simulink model "SF012A_HysCmp"  (R2013b)
settings: Solver=FixedStepDiscrete  StartTime=0.0  StopTime=1  FixedStep=.002  RelTol=1e-3
values from neighbouring files (symbols this model uses):
  ARCHGLBPRM_2MILLISEC_SEC_F32 = DataDict.Constant    [SF012A_HysCmp_DataDict.m]
  EPSILON_ULS_F32 = DataDict.Constant    [SF012A_HysCmp_DataDict.m]
  FLTINJ_HYSCMP_HYSCMPCMD = DataDict.Constant    [SF012A_HysCmp_DataDict.m]
  HysCmpAssiInpLim = DataDict.Calibration    [SF012A_HysCmp_DataDict.m]
  HysCmpOutpLim = DataDict.Calibration    [SF012A_HysCmp_DataDict.m]
  HysCmpRevGain = DataDict.Calibration    [SF012A_HysCmp_DataDict.m]
  HysCmpRiseX = DataDict.Calibration    [SF012A_HysCmp_DataDict.m]
  HysCmpRiseY = DataDict.Calibration    [SF012A_HysCmp_DataDict.m]
  HYSRISEYLIM_ULS_F32 = DataDict.Constant    [SF012A_HysCmp_DataDict.m]
  HYSSATNLOWLIM_HWNWTMTR_F32 = DataDict.Constant    [SF012A_HysCmp_DataDict.m]
  SysGlbPrmSysTqRat = DataDict.ImprtdCal    [SF012A_HysCmp_DataDict.m]
libraries: FixdToFloat x18, FloatToFixd x14, LnrIntrpn x12, NxtrAbslt x10, NxtrLim x8, Fil x6, NxtrSign x5, simulink x2, NxtrMath x1, BilnrIntrpnMplX x1, NxtrMax x1
(part 1 of 3)
settings Model: Creator=TZ5743  LastModifiedBy=NZ2883
settings DataIOCC: LimitDataPoints=off  SaveFormat=Structure  ReturnWorkspaceOutputs=on
settings OptimizationCC: BlockReduction=off  InlineParams=on  ZeroExternalMemoryAtStartup=off  ZeroInternalMemoryAtStartup=off  OptimizeModelRefInitCode=on  LifeSpan=1
settings DebuggingCC: SignalInfNanChecking=error  SignalRangeChecking=warning  UnderspecifiedInitializationDetection=Simplified  SolverPrmCheckMsg=error  InheritedTsInSrcMsg=error  DiscreteInheritContinuousMsg=error  SingleTaskRateTransMsg=error  TasksWithSamePriorityMsg=error  SigSpecEnsureSampleTimeMsg=error  CheckMatrixSingularityMsg=error  IntegerOverflowMsg=error  ParameterUnderflowMsg=error  ParameterPrecisionLossMsg=error  ParameterTunabilityLossMsg=error  FixptConstUnderflowMsg=warning  FixptConstOverflowMsg=warning  VectorMatrixConversionMsg=error  SignalLabelMismatchMsg=error  UnconnectedInputMsg=error  UnconnectedOutputMsg=error  UnconnectedLineMsg=error  SFcnCompatibilityMsg=error  UniqueDataStoreMsg=warning  BusObjectLabelMismatch=error  RootOutportRequireBusObject=error  AssertControl=DisableAll  ModelReferenceIOMsg=error  ModelReferenceVersionMismatchMessage=warning  ModelReferenceIOMismatchMessage=error  ModelReferenceCSMismatchMessage=warning  ModelReferenceDataLoggingMessage=error  StateNameClashWarn=warning  StrictBusMsg=ErrorOnBusTreatedAsVector  NonBusSignalsTreatedAsBus=error  SFUnexpectedBacktrackingDiag=error  SFInvalidInputDataAccessInChartInitDiag=error  SFNoUnconditionalDefaultTransitionDiag=error  SFTransitionOutsideNaturalParentDiag=error  SFUnconditionalTransitionShadowingDiag=error  SFUndirectedBroadcastEventsDiag=error
settings ModelReferenceCC: ModelReferenceNumInstancesAllowed=Single
settings RTWCC: SystemTargetFile=autosar.tlc  GenCodeOnly=on  TemplateMakefile=ert_default_tmf  Description=AUTOSAR  GenerateReport=on  ProcessScript=autosar_make_rtw_hook  LaunchReport=on
settings CodeAppCC: GenerateComments=off  IgnoreCustomStorageClasses=off  CustomSymbolStrType=$N$R$M  CustomSymbolStrBlkIO=$N$M  SimulinkBlockComments=off
settings STFCustomTargetCC: ParMdlRefBuildCompliant=on  CompOptLevelCompliant=on  IncludeMdlTerminateFcn=off  CombineOutputUpdateFcns=on  SuppressErrorStatus=on  ERTFirstTimeCompliant=on  ERTCustomFileBanners=on  SupportNonFinite=off  SupportComplex=off  SupportContinuousTime=off  SupportNonInlinedSFcns=off  MATLABClassNameForMDSCustomization=Simulink.SoftwareTarget.ERTCustomization  AutosarCompliant=on  GRTInterface=off  SystemTargetFile=autosar.tlc
settings ERTTargetCC: CodeReplacementLibrary=ANSI_C  ConcurrentExecutionCompliant=off  IncludeMdlTerminateFcn=off  SuppressErrorStatus=on  SupportNonFinite=off  SupportComplex=off  ModelStepFunctionPrototypeControlCompliant=off  CPPClassGenCompliant=off  AutosarCompliant=on  InlinedParameterPlacement=NonHierarchical  ERTCustomFileTemplate=example_file_process.tlc  EnableUserReplacementTypes=on

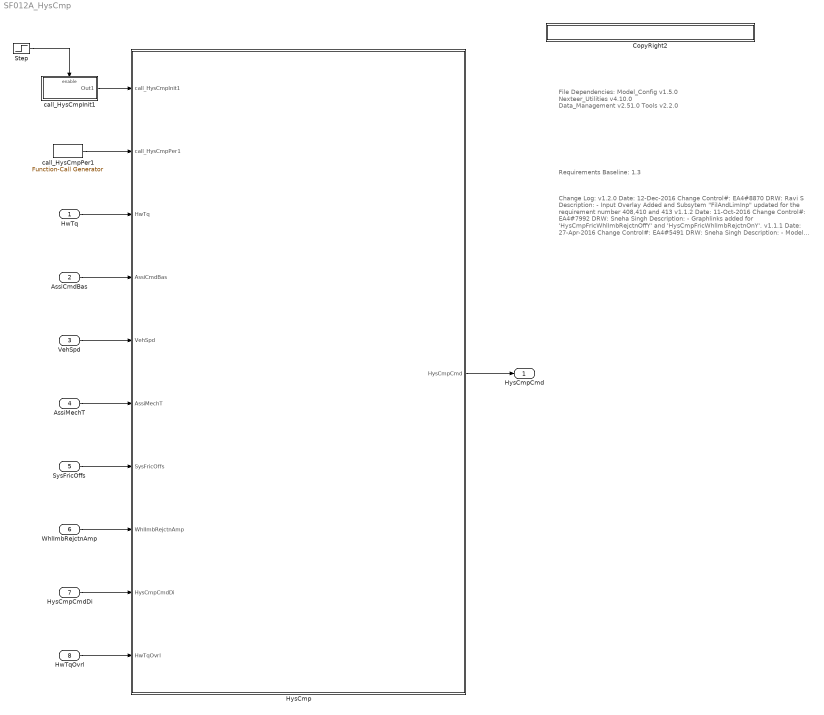
== system SF012A_HysCmp ==
  note: File Dependencies:
      |
      | Model_Config v1.5.0
      | Nexteer_Utilities v4.10.0
      | Data_Management v2.51.0
      | Tools v2.2.0
  note: Requirements Baseline: 1.3
  note: Change Log:
      |
      | v1.2.0
      | Date: 12-Dec-2016
      | Change Control#: EA4#8870
      | DRW: Ravi S
      | Description:
      | - Input Overlay Added and Subsytem "FilAndLimInp" updated
      |  for the requirement number 408,410 and 413
      |
      | v1.1.2
      | Date: 11-Oct-2016
      | Change Control#: EA4#7992
      | DRW: Sneha Singh
      | Description:
      | - Graphlinks added for 'HysCmpFricWhlImbRejctnOffY'
      | and 'HysCmpFricWhlImbRejctnOnY'.
      |
      | v1.1.1
      | Date: 27-Apr-2016
      | Change Control#: EA4#5491
      | DRW: Sneha Singh
      | Description:
      | - Model traceability performed in DOORS.
      |
      | v1.1.0
      | Date: 24-DEC-2015
      | Change Control #: EA4#2177
      | DRW:  Sumit/Muragesh(KPIT)
      | Description:
      | -  LPF block kept outside IF/ELSE Blocks from HysCmp.
      |
      | v1.0.0
      | Date: 08-Jul-2015
      | Change Control #: EA4#943
      | Author:  Sudeep Shankar
      | Description:
      | - Initial Release based off of EA3 Version 008
  HwTq : Inport  RequirementInfo={'linktype_rmi_doors' '0000a52c (/E-STEER Core/SubSystem Specifications/Application Functions/SF012A Hysteresis Compensation)' '#SF012A_393' 'true' 'REQ:SF012A_393' '' } %GIDa_39e8ddae_593d_4cef_93cb_543cdb158812
  AssiCmdBas : Inport  RequirementInfo={'linktype_rmi_doors' '0000a52c (/E-STEER Core/SubSystem Specifications/Application Functions/SF012A Hysteresis Compensation)' '#SF012A_394' 'true' 'REQ:SF012A_394' '' } %GIDa_43c2c86b_c386_4b36_8120_f78d8358a699  Port=2
  VehSpd : Inport  RequirementInfo={'linktype_rmi_doors' '0000a52c (/E-STEER Core/SubSystem Specifications/Application Functions/SF012A Hysteresis Compensation)' '#SF012A_395' 'true' 'REQ:SF012A_395' '' } %GIDa_41cfc9f5_b645_48be_a67a_9b819ba6b5fb  Port=3
  AssiMechT : Inport  RequirementInfo={'linktype_rmi_doors' '0000a52c (/E-STEER Core/SubSystem Specifications/Application Functions/SF012A Hysteresis Compensation)' '#SF012A_396' 'true' 'REQ:SF012A_396' '' } %GIDa_4288aa5f_4c37_4962_8431_89a584e38b5d  Port=4
  SysFricOffs : Inport  RequirementInfo={'linktype_rmi_doors' '0000a52c (/E-STEER Core/SubSystem Specifications/Application Functions/SF012A Hysteresis Compensation)' '#SF012A_397' 'true' 'REQ:SF012A_397' '' } %GIDa_af008a60_1b2d_4e4c_829a_d9cddebe7ac0  Port=5
  WhlImbRejctnAmp : Inport  RequirementInfo={'linktype_rmi_doors' '0000a52c (/E-STEER Core/SubSystem Specifications/Application Functions/SF012A Hysteresis Compensation)' '#SF012A_398' 'true' 'REQ:SF012A_398' '' } %GIDa_233b884d_e34c_40db_ae2f_04f6db5d5afb  Port=6
  HysCmpCmdDi : Inport  RequirementInfo={'linktype_rmi_doors' '0000a52c (/E-STEER Core/SubSystem Specifications/Application Functions/SF012A Hysteresis Compensation)' '#SF012A_399' 'true' 'REQ:SF012A_399' '' } %GIDa_f4b38744_58c4_4286_8088_54ff54dead4c  Port=7
  HwTqOvrl : Inport  RequirementInfo="{'linktype_rmi_doors' '0000a52c (/E-STEER Core/SubSystem Specifications/Application Functions/SF012A Hysteresis Compensation)' '#SF012A_488' 'true' 'REQ:  SF012A_488' '' } %GIDa_12de40c4_b1ed_4f19_94f5_63d2f2c5e810"  Port=8
  CopyRight2 : Subsystem  Description=|  mask(Copyright Information){none=on}
      | Copyright info block.                                               
      |                                                                     
      | Place copyright information at the top of every subsystem in design.
      mask prompts: none "No parameters"
      mask help: Place copyright information at the top of every subsystem in design.
      mask Display:
      | NxtrConf = 'Nexteer Confidential';
      | 
      | sys = bdroot; %handle for the current model ("system")
      | first = get_param(sys,'Created');
      | if(isempty(first))
      |     first = datestr(now,'yyyy');
      | else
      |     first = first(end-3:end);  %year is last four digits
      | end
      | 
      | last = get_param(sys,'LastModifiedDate');
      | if isempty(last)
      |     last = datestr(now,'yyyy');
      | else
      |     last = last(end-3:end);
      | end
      | 
      | if strcmp(first,last)
      |     fprintf('%s -- Copyright %s Nexteer',NxtrConf,first)
      | else
      |     fprintf('%s -- %s%s- %s Nexteer',NxtrConf,char(169),first,last)
      | end
  HysCmp : Subsystem
  Step : Step  Time=.001  Before=1  After=0  SampleTime=0
  call_HysCmpInit1 : Subsystem  TreatAsAtomicUnit=on
  call_HysCmpPer1 : simulink/Ports & Subsystems/Function-Call Generator  RequirementInfo={'linktype_rmi_doors' '0000a52c (/E-STEER Core/SubSystem Specifications/Application Functions/SF012A Hysteresis Compensation)' '#SF012A_469' 'true' 'REQ:SF012A_469' '' } %GIDa_211e4458_5e3d_455a_8408_cf5f2d6f0325  sample_time=0.002  numberOfIterations=1
  HysCmpCmd : Outport  RequirementInfo={'linktype_rmi_doors' '0000a52c (/E-STEER Core/SubSystem Specifications/Application Functions/SF012A Hysteresis Compensation)' '#SF012A_401' 'true' 'REQ:SF012A_401' '' } %GIDa_f3032a14_e69b_4692_8266_2bd5cb5a9d4b
  wires:
  HwTq/1 -> HysCmp/3(HwTq)
  AssiCmdBas/1 -> HysCmp/4(AssiCmdBas)
  VehSpd/1 -> HysCmp/5(VehSpd)
  AssiMechT/1 -> HysCmp/6(AssiMechT)
  SysFricOffs/1 -> HysCmp/7(SysFricOffs)
  WhlImbRejctnAmp/1 -> HysCmp/8(WhlImbRejctnAmp)
  HysCmpCmdDi/1 -> HysCmp/9(HysCmpCmdDi)
  HysCmp/1(HysCmpCmd) -> HysCmpCmd/1
  call_HysCmpPer1/1 -> HysCmp/2(call_HysCmpPer1)
  call_HysCmpInit1/1(Out1) -> HysCmp/1(call_HysCmpInit1)
  Step/1 -> call_HysCmpInit1/Enable
  HwTqOvrl/1 -> HysCmp/10(HwTqOvrl)

== system SF012A_HysCmp/CopyRight2 ==

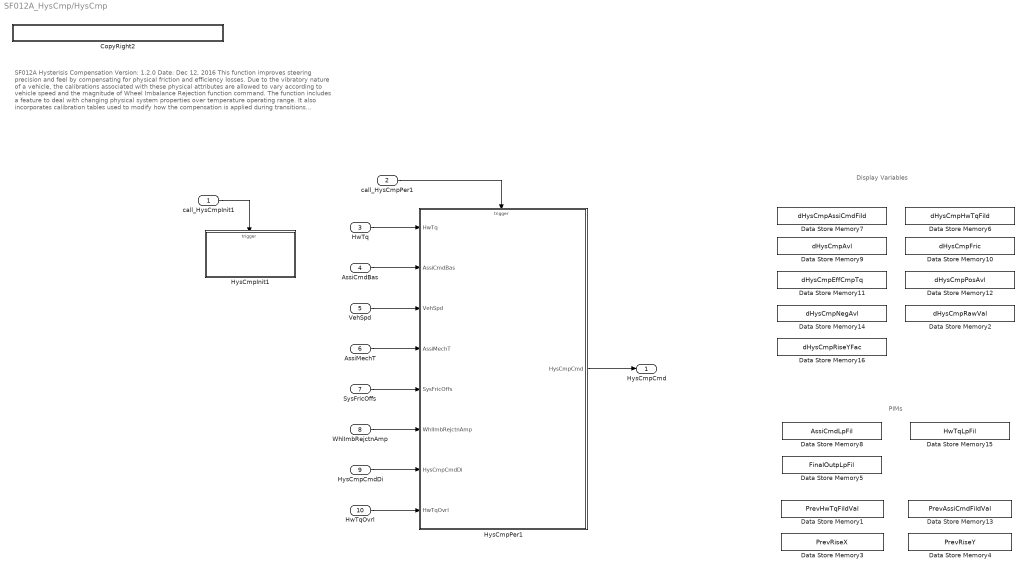
== system SF012A_HysCmp/HysCmp ==
  note: SF012A Hysterisis Compensation       Version: 1.2.0                                                      Date: Dec 12, 2016
      |
      | This function improves steering precision and feel by compensating for physical friction and efficiency losses.
      | Due to the vibratory nature of a vehicle, the calibrations associated with these physical attributes are allowed
      | to vary according to vehicle speed and the magnitude of Wheel Imbalance Rejection function command. The function
      | includes a feature to deal with changing physical system properties over temperature operating range. It also
      | incorporates calibration tables used to modify how the compensation is applied during transitions between operating
      | quadrants and during periods of near-zero handwheel torque. Finally the function may be disabled for purposes of
      | bench testing
  note: PIMs
  note: Display Variables
  call_HysCmpInit1 : Inport
  call_HysCmpPer1 : Inport  Port=2
  HwTq : Inport  Port=3
  AssiCmdBas : Inport  Port=4
  VehSpd : Inport  Port=5
  AssiMechT : Inport  Port=6
  SysFricOffs : Inport  Port=7
  WhlImbRejctnAmp : Inport  Port=8
  HysCmpCmdDi : Inport  Port=9
  HwTqOvrl : Inport  RequirementInfo={} %GIDa_ad37b2a9_b40c_4d54_905f_1c586e369e0d  Port=10
  CopyRight2 : Subsystem  Description=|  mask(Copyright Information){none=on}
      | Copyright info block.                                               
      |                                                                     
      | Place copyright information at the top of every subsystem in design.
      mask prompts: none "No parameters"
      mask help: Place copyright information at the top of every subsystem in design.
      mask Display:
      | NxtrConf = 'Nexteer Confidential';
      | 
      | sys = bdroot; %handle for the current model ("system")
      | first = get_param(sys,'Created');
      | if(isempty(first))
      |     first = datestr(now,'yyyy');
      | else
      |     first = first(end-3:end);  %year is last four digits
      | end
      | 
      | last = get_param(sys,'LastModifiedDate');
      | if isempty(last)
      |     last = datestr(now,'yyyy');
      | else
      |     last = last(end-3:end);
      | end
      | 
      | if strcmp(first,last)
      |     fprintf('%s -- Copyright %s Nexteer',NxtrConf,first)
      | else
      |     fprintf('%s -- %s%s- %s Nexteer',NxtrConf,char(169),first,last)
      | end
  Data Store Memory1 : DataStoreMemory  DataStoreName=PrevHwTqFildVal  StateMustResolveToSignalObject=on
  Data Store Memory10 : DataStoreMemory  DataStoreName=dHysCmpFric  ReadBeforeWriteMsg=warning  WriteAfterWriteMsg=warning  WriteAfterReadMsg=warning  StateMustResolveToSignalObject=on
  Data Store Memory11 : DataStoreMemory  DataStoreName=dHysCmpEffCmpTq  ReadBeforeWriteMsg=warning  WriteAfterWriteMsg=warning  WriteAfterReadMsg=warning  StateMustResolveToSignalObject=on
  Data Store Memory12 : DataStoreMemory  DataStoreName=dHysCmpPosAvl  ReadBeforeWriteMsg=warning  WriteAfterWriteMsg=warning  WriteAfterReadMsg=warning  StateMustResolveToSignalObject=on
  Data Store Memory13 : DataStoreMemory  DataStoreName=PrevAssiCmdFildVal  StateMustResolveToSignalObject=on
  Data Store Memory14 : DataStoreMemory  DataStoreName=dHysCmpNegAvl  ReadBeforeWriteMsg=warning  WriteAfterWriteMsg=warning  WriteAfterReadMsg=warning  StateMustResolveToSignalObject=on
  Data Store Memory15 : DataStoreMemory  DataStoreName=HwTqLpFil  InitialValue=struct('FilSt',single(0),'FilGain',single(0))  OutDataTypeStr=Bus: FilLpRec1  StateMustResolveToSignalObject=on
  Data Store Memory16 : DataStoreMemory  DataStoreName=dHysCmpRiseYFac  ReadBeforeWriteMsg=warning  WriteAfterWriteMsg=warning  WriteAfterReadMsg=warning  StateMustResolveToSignalObject=on
  Data Store Memory2 : DataStoreMemory  DataStoreName=dHysCmpRawVal  ReadBeforeWriteMsg=warning  WriteAfterWriteMsg=warning  WriteAfterReadMsg=warning  StateMustResolveToSignalObject=on
  Data Store Memory3 : DataStoreMemory  DataStoreName=PrevRiseX  StateMustResolveToSignalObject=on
  Data Store Memory4 : DataStoreMemory  DataStoreName=PrevRiseY  StateMustResolveToSignalObject=on
  Data Store Memory5 : DataStoreMemory  DataStoreName=FinalOutpLpFil  InitialValue=struct('FilSt',single(0),'FilGain',single(0))  OutDataTypeStr=Bus: FilLpRec1  StateMustResolveToSignalObject=on
  Data Store Memory6 : DataStoreMemory  DataStoreName=dHysCmpHwTqFild  ReadBeforeWriteMsg=warning  WriteAfterWriteMsg=warning  WriteAfterReadMsg=warning  StateMustResolveToSignalObject=on
  Data Store Memory7 : DataStoreMemory  DataStoreName=dHysCmpAssiCmdFild  ReadBeforeWriteMsg=warning  WriteAfterWriteMsg=warning  WriteAfterReadMsg=warning  StateMustResolveToSignalObject=on
  Data Store Memory8 : DataStoreMemory  DataStoreName=AssiCmdLpFil  InitialValue=struct('FilSt',single(0),'FilGain',single(0))  OutDataTypeStr=Bus: FilLpRec1  StateMustResolveToSignalObject=on
  Data Store Memory9 : DataStoreMemory  DataStoreName=dHysCmpAvl  ReadBeforeWriteMsg=warning  WriteAfterWriteMsg=warning  WriteAfterReadMsg=warning  StateMustResolveToSignalObject=on
  HysCmpInit1 : Subsystem
  HysCmpPer1 : Subsystem
  HysCmpCmd : Outport
  wires:
  call_HysCmpInit1/1 -> HysCmpInit1/Trigger
  HwTq/1 -> HysCmpPer1/1(HwTq)
  AssiCmdBas/1 -> HysCmpPer1/2(AssiCmdBas)
  call_HysCmpPer1/1 -> HysCmpPer1/Trigger
  HysCmpPer1/1(HysCmpCmd) -> HysCmpCmd/1
  VehSpd/1 -> HysCmpPer1/3(VehSpd)
  AssiMechT/1 -> HysCmpPer1/4(AssiMechT)
  SysFricOffs/1 -> HysCmpPer1/5(SysFricOffs)
  WhlImbRejctnAmp/1 -> HysCmpPer1/6(WhlImbRejctnAmp)
  HysCmpCmdDi/1 -> HysCmpPer1/7(HysCmpCmdDi)
  HwTqOvrl/1 -> HysCmpPer1/8(HwTqOvrl)

== system SF012A_HysCmp/call_HysCmpInit1 ==
  Enable : EnablePort
  Function-Call Generator : simulink/Ports & Subsystems/Function-Call Generator  sample_time=.002  numberOfIterations=1
  Out1 : Outport
  wires:
  Function-Call Generator/1 -> Out1/1

== system SF012A_HysCmp/HysCmp/CopyRight2 ==

== system SF012A_HysCmp/HysCmp/HysCmpInit1 ==
  function : TriggerPort  TriggerType=function-call
  CopyRight2 : Subsystem  Description=|  mask(Copyright Information){none=on}
      | Copyright info block.                                               
      |                                                                     
      | Place copyright information at the top of every subsystem in design.
      mask prompts: none "No parameters"
      mask help: Place copyright information at the top of every subsystem in design.
      mask Display:
      | NxtrConf = 'Nexteer Confidential';
      | 
      | sys = bdroot; %handle for the current model ("system")
      | first = get_param(sys,'Created');
      | if(isempty(first))
      |     first = datestr(now,'yyyy');
      | else
      |     first = first(end-3:end);  %year is last four digits
      | end
      | 
      | last = get_param(sys,'LastModifiedDate');
      | if isempty(last)
      |     last = datestr(now,'yyyy');
      | else
      |     last = last(end-3:end);
      | end
      | 
      | if strcmp(first,last)
      |     fprintf('%s -- Copyright %s Nexteer',NxtrConf,first)
      | else
      |     fprintf('%s -- %s%s- %s Nexteer',NxtrConf,char(169),first,last)
      | end
  HysCmpAssiCmdLpFilInit1 : Fil/FilLpInit  Ic=0  Ts=ARCHGLBPRM_2MILLISEC_SEC_F32  Freq=HysCmpAssiCmdLpFilFrq  StVar=AssiCmdLpFil
  HysCmpFinalOutpLpFil1 : Fil/FilLpInit  Ic=0  Ts=ARCHGLBPRM_2MILLISEC_SEC_F32  Freq=HysCmpFinalOutpLpFilFrq  StVar=FinalOutpLpFil
  HysCmpHwTqLpFilInit : Fil/FilLpInit  Ic=0  Ts=ARCHGLBPRM_2MILLISEC_SEC_F32  Freq=HysCmpHwTqLpFilFrq  StVar=HwTqLpFil

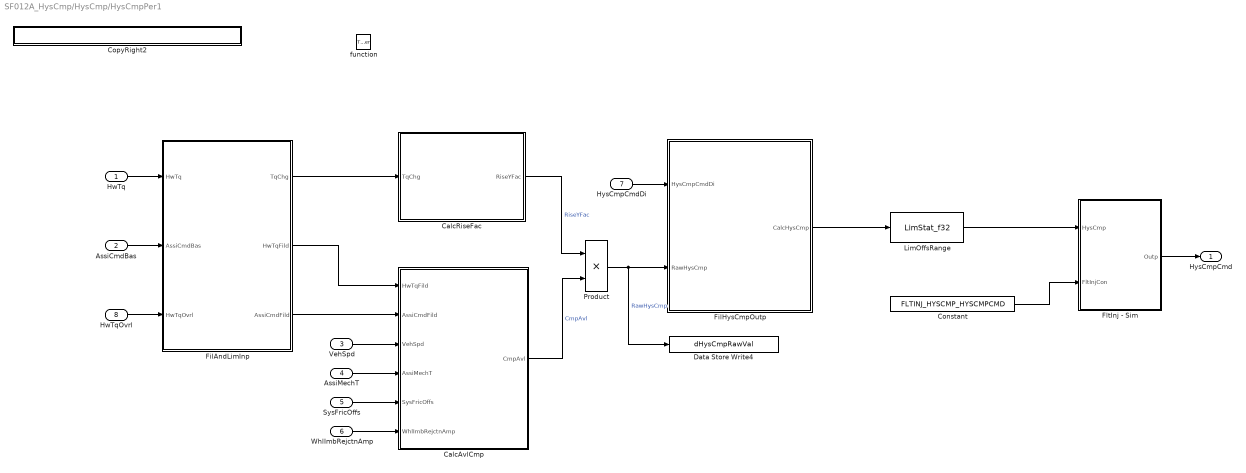
== system SF012A_HysCmp/HysCmp/HysCmpPer1 ==
  HwTq : Inport
  AssiCmdBas : Inport  Port=2
  VehSpd : Inport  Port=3
  AssiMechT : Inport  Port=4
  SysFricOffs : Inport  Port=5
  WhlImbRejctnAmp : Inport  Port=6
  HysCmpCmdDi : Inport  Port=7
  HwTqOvrl : Inport  RequirementInfo={} %GIDa_e9591222_eece_4b59_ae76_baf43c703f32  Port=8
  function : TriggerPort  TriggerType=function-call
  CalcAvlCmp : Subsystem  RequirementInfo={'linktype_rmi_doors' '0000a52c (/E-STEER Core/SubSystem Specifications/Application Functions/SF012A Hysteresis Compensation)' '#SF012A_437' 'true' 'REQ:SF012A_437' '' } %GIDa_e1ddb5a7_9fd6_44f0_bdf5_870e145ff722
  CalcRiseFac : Subsystem
  Constant : Constant  Value=FLTINJ_HYSCMP_HYSCMPCMD
  CopyRight2 : Subsystem  Description=|  mask(Copyright Information){none=on}
      | Copyright info block.                                               
      |                                                                     
      | Place copyright information at the top of every subsystem in design.
      mask prompts: none "No parameters"
      mask help: Place copyright information at the top of every subsystem in design.
      mask Display:
      | NxtrConf = 'Nexteer Confidential';
      | 
      | sys = bdroot; %handle for the current model ("system")
      | first = get_param(sys,'Created');
      | if(isempty(first))
      |     first = datestr(now,'yyyy');
      | else
      |     first = first(end-3:end);  %year is last four digits
      | end
      | 
      | last = get_param(sys,'LastModifiedDate');
      | if isempty(last)
      |     last = datestr(now,'yyyy');
      | else
      |     last = last(end-3:end);
      | end
      | 
      | if strcmp(first,last)
      |     fprintf('%s -- Copyright %s Nexteer',NxtrConf,first)
      | else
      |     fprintf('%s -- %s%s- %s Nexteer',NxtrConf,char(169),first,last)
      | end
  Data Store Write4 : DataStoreWrite  DataStoreName=dHysCmpRawVal
  FilAndLimInp : Subsystem
  FilHysCmpOutp : Subsystem  RequirementInfo={'linktype_rmi_doors' '0000a52c (/E-STEER Core/SubSystem Specifications/Application Functions/SF012A Hysteresis Compensation)' '#SF012A_455' 'true' 'REQ:SF012A_455' '' } %GIDa_f9dc65f2_b670_4a31_9af7_0f46f3c3f7f0
  FltInj - Sim : Subsystem  RequirementInfo={'linktype_rmi_doors' '0000a52c (/E-STEER Core/SubSystem Specifications/Application Functions/SF012A Hysteresis Compensation)' '#SF012A_472' 'true' 'REQ:SF012A_472' '' } %GIDa_a7a86232_8456_4bcb_93e6_5959b283ff17  TreatAsAtomicUnit=on  VariantControl=FltInj_sim  mask(Fault_Injection){}
      mask help: Fault Injection is a simulation only block for EA4 programs.
  LimOffsRange : NxtrLim/LimStat_f32  RequirementInfo={'linktype_rmi_doors' '0000a52c (/E-STEER Core/SubSystem Specifications/Application Functions/SF012A Hysteresis Compensation)' '#SF012A_460' 'true' 'REQ:SF012A_460' '' ; 'linktype_rmi_doors' '0000a52c (/E-STEER Core/SubSystem Specifications/Application Functions/SF012A Hysteresis Compensation)' '#SF012A_465' 'true' 'REQ:SF012A_465' '' } %GIDa_90a5b817_40fa_4bb3_abf4_98fe238a427b  LoLim=SYSGLBPRM_MOTTQCMDLOLIM_MOTNWTMTR_F32  HiLim=SYSGLBPRM_MOTTQCMDHILIM_MOTNWTMTR_F32
      settings: AttributesFormatString=|
      | Low Limit: %<LoLim>
      | High Limit:%<HiLim>
  Product : Product  RequirementInfo={'linktype_rmi_doors' '0000a52c (/E-STEER Core/SubSystem Specifications/Application Functions/SF012A Hysteresis Compensation)' '#SF012A_456' 'true' 'REQ:SF012A_456' '' } %GIDa_0302521d_8ef1_4311_9c92_13702153adce  OutDataTypeStr=Inherit: Inherit via back propagation  RndMeth=Zero
  HysCmpCmd : Outport  RequirementInfo={'linktype_rmi_doors' '0000a52c (/E-STEER Core/SubSystem Specifications/Application Functions/SF012A Hysteresis Compensation)' '#SF012A_458' 'true' 'REQ:SF012A_458' '' } %GIDa_7cd43374_63d5_4d88_b8d5_6926c5b73d3e
  wires:
  HwTq/1 -> FilAndLimInp/1(HwTq)
  AssiCmdBas/1 -> FilAndLimInp/2(AssiCmdBas)
  FilAndLimInp/3(AssiCmdFild) -> CalcAvlCmp/2(AssiCmdFild)
  FilAndLimInp/1(TqChg) -> CalcRiseFac/1(TqChg)
  FilAndLimInp/2(HwTqFild) -> CalcAvlCmp/1(HwTqFild)
  SysFricOffs/1 -> CalcAvlCmp/5(SysFricOffs)
  AssiMechT/1 -> CalcAvlCmp/4(AssiMechT)
  VehSpd/1 -> CalcAvlCmp/3(VehSpd)
  WhlImbRejctnAmp/1 -> CalcAvlCmp/6(WhlImbRejctnAmp)
  CalcRiseFac/1(RiseYFac) -> Product/1  "RiseYFac"
  CalcAvlCmp/1(CmpAvl) -> Product/2  "CmpAvl"
  Product/1 -> FilHysCmpOutp/2(RawHysCmp), Data Store Write4/1  "RawHysCmp"
  HysCmpCmdDi/1 -> FilHysCmpOutp/1(HysCmpCmdDi)
  FilHysCmpOutp/1(CalcHysCmp) -> LimOffsRange/1
  Constant/1 -> FltInj - Sim/2(FltInjCon)
  FltInj - Sim/1(Outp) -> HysCmpCmd/1
  LimOffsRange/1 -> FltInj - Sim/1(HysCmp)
  HwTqOvrl/1 -> FilAndLimInp/3(HwTqOvrl)

== system SF012A_HysCmp/HysCmp/HysCmpInit1/CopyRight2 ==

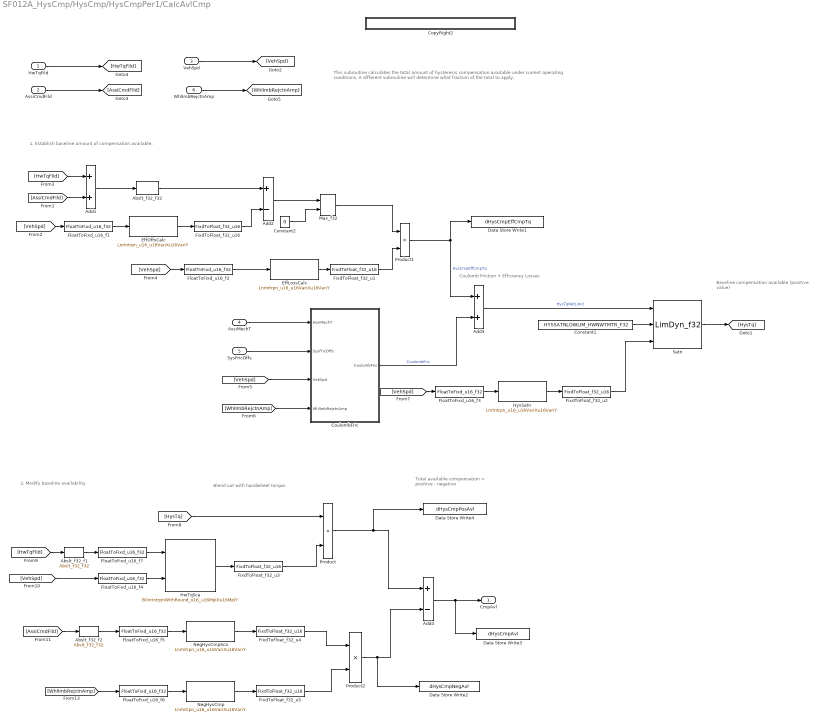
== system SF012A_HysCmp/HysCmp/HysCmpPer1/CalcAvlCmp ==
  note: This subroutine calculates the total amount of hysteresis compensation available under current operating conditions.
      | A different subroutine will determine what fraction of the total to apply.
  note: Total available compensation
      | = positive - negative
  note: Blend out with handwheel torque.
  note: 2. Modify baseline availability
  note: 1. Establish baseline amount of compensation available.
  note: Baseline compensation available
      | (positive value)
  note: Coulomb Friction + Efficiency Losses
  HwTqFild : Inport
  AssiCmdFild : Inport  Port=2
  VehSpd : Inport  Port=3
  AssiMechT : Inport  Port=4
  SysFricOffs : Inport  Port=5
  WhlImbRejctnAmp : Inport  Port=6
  Abslt_f32_f1 : NxtrAbslt/Abslt_f32_f32  RequirementInfo={'linktype_rmi_doors' '0000a52c (/E-STEER Core/SubSystem Specifications/Application Functions/SF012A Hysteresis Compensation)' '#SF012A_452' 'true' 'REQ:SF012A_452' '' } %GIDa_d0e45d04_1280_4e0b_943d_6041d06ef4f5  SFunctionSpec=single y1 = Abslt_f32_f32(single u1)
      settings: AttributesFormatString=%<Name>
  Abslt_f32_f2 : NxtrAbslt/Abslt_f32_f32  RequirementInfo={'linktype_rmi_doors' '0000a52c (/E-STEER Core/SubSystem Specifications/Application Functions/SF012A Hysteresis Compensation)' '#SF012A_453' 'true' 'REQ:SF012A_453' '' } %GIDa_1bd873dd_78ad_4665_a6ac_86e46d9a2c21  SFunctionSpec=single y1 = Abslt_f32_f32(single u1)
      settings: AttributesFormatString=%<Name>
  Abslt_f32_f32 : NxtrAbslt/Abslt_f32_f32  RequirementInfo={'linktype_rmi_doors' '0000a52c (/E-STEER Core/SubSystem Specifications/Application Functions/SF012A Hysteresis Compensation)' '#SF012A_442' 'true' 'REQ:SF012A_442' '' } %GIDa_abee7619_0beb_4c1e_8921_36a91baf6c7f  SFunctionSpec=single y1 = Abslt_f32_f32(single u1)
      settings: AttributesFormatString=%<Name>
  Add1 : Sum  RequirementInfo={'linktype_rmi_doors' '0000a52c (/E-STEER Core/SubSystem Specifications/Application Functions/SF012A Hysteresis Compensation)' '#SF012A_442' 'true' 'REQ:SF012A_442' '' } %GIDa_bfcac00b_6b92_41b4_8339_9aa0e2e33000  RndMeth=Zero
  Add2 : Sum  RequirementInfo={'linktype_rmi_doors' '0000a52c (/E-STEER Core/SubSystem Specifications/Application Functions/SF012A Hysteresis Compensation)' '#SF012A_442' 'true' 'REQ:SF012A_442' '' } %GIDa_2295aae0_36c4_422f_b656_25e81def27bc  Inputs=+-  RndMeth=Zero
  Add3 : Sum  RequirementInfo={'linktype_rmi_doors' '0000a52c (/E-STEER Core/SubSystem Specifications/Application Functions/SF012A Hysteresis Compensation)' '#SF012A_439' 'true' 'REQ:SF012A_439' '' } %GIDa_7fe7bab0_9e12_422c_a564_b3e8ab419555  RndMeth=Zero
  Add4 : Sum  RequirementInfo={'linktype_rmi_doors' '0000a52c (/E-STEER Core/SubSystem Specifications/Application Functions/SF012A Hysteresis Compensation)' '#SF012A_454' 'true' 'REQ:SF012A_454' '' } %GIDa_3a6b5736_20ef_483b_bd10_13c84a375067  Inputs=+-  RndMeth=Zero
  Constant1 : Constant  RequirementInfo={'linktype_rmi_doors' '0000a52c (/E-STEER Core/SubSystem Specifications/Application Functions/SF012A Hysteresis Compensation)' '#SF012A_440' 'true' 'REQ:SF012A_440' '' } %GIDa_72c8f7eb_1423_42d2_b600_2953d8412076  Value=HYSSATNLOWLIM_HWNWTMTR_F32
  Constant2 : Constant  RequirementInfo={'linktype_rmi_doors' '0000a52c (/E-STEER Core/SubSystem Specifications/Application Functions/SF012A Hysteresis Compensation)' '#SF012A_442' 'true' 'REQ:SF012A_442' '' } %GIDa_4f4bccf0_dacb_4e1d_ba24_65729ec75eb9  Value=0  OutDataTypeStr=single
  CopyRight2 : Subsystem  Description=|  mask(Copyright Information){none=on}
      | Copyright info block.                                               
      |                                                                     
      | Place copyright information at the top of every subsystem in design.
      mask prompts: none "No parameters"
      mask help: Place copyright information at the top of every subsystem in design.
      mask Display:
      | NxtrConf = 'Nexteer Confidential';
      | 
      | sys = bdroot; %handle for the current model ("system")
      | first = get_param(sys,'Created');
      | if(isempty(first))
      |     first = datestr(now,'yyyy');
      | else
      |     first = first(end-3:end);  %year is last four digits
      | end
      | 
      | last = get_param(sys,'LastModifiedDate');
      | if isempty(last)
      |     last = datestr(now,'yyyy');
      | else
      |     last = last(end-3:end);
      | end
      | 
      | if strcmp(first,last)
      |     fprintf('%s -- Copyright %s Nexteer',NxtrConf,first)
      | else
      |     fprintf('%s -- %s%s- %s Nexteer',NxtrConf,char(169),first,last)
      | end
  CoulombFric : Subsystem  RequirementInfo={'linktype_rmi_doors' '0000a52c (/E-STEER Core/SubSystem Specifications/Application Functions/SF012A Hysteresis Compensation)' '#SF012A_444' 'true' 'REQ:SF012A_444' '' } %GIDa_833fc1c6_1365_47d5_a369_624d6f944246
  Data Store Write1 : DataStoreWrite  RequirementInfo={'linktype_rmi_doors' '0000a52c (/E-STEER Core/SubSystem Specifications/Application Functions/SF012A Hysteresis Compensation)' '#SF012A_441' 'true' 'REQ:SF012A_441' '' } %GIDa_2a47f852_9866_4d0e_b49b_3a819b376f8e  DataStoreName=dHysCmpEffCmpTq
  Data Store Write2 : DataStoreWrite  RequirementInfo={'linktype_rmi_doors' '0000a52c (/E-STEER Core/SubSystem Specifications/Application Functions/SF012A Hysteresis Compensation)' '#SF012A_453' 'true' 'REQ:SF012A_453' '' } %GIDa_0b356355_9b93_41f9_90a1_a7e73be94b81  DataStoreName=dHysCmpNegAvl
  Data Store Write3 : DataStoreWrite  RequirementInfo={'linktype_rmi_doors' '0000a52c (/E-STEER Core/SubSystem Specifications/Application Functions/SF012A Hysteresis Compensation)' '#SF012A_454' 'true' 'REQ:SF012A_454' '' } %GIDa_edc36cc5_35db_4e88_a6bf_d23be94f94f4  DataStoreName=dHysCmpAvl
  Data Store Write4 : DataStoreWrite  RequirementInfo={'linktype_rmi_doors' '0000a52c (/E-STEER Core/SubSystem Specifications/Application Functions/SF012A Hysteresis Compensation)' '#SF012A_452' 'true' 'REQ:SF012A_452' '' } %GIDa_082867ec_9786_4d8c_ad02_ca886b84261e  DataStoreName=dHysCmpPosAvl
  EffLossCalc : LnrIntrpn/LnrIntrpn_u16_u16VariXu16VariY  RequirementInfo={'linktype_rmi_doors' '0000a52c (/E-STEER Core/SubSystem Specifications/Application Functions/SF012A Hysteresis Compensation)' '#SF012A_443' 'true' 'REQ:SF012A_443' '' } %GIDa_8df0684c_85cd_4686_a96d_1bf52a3859b7  XTbl=SysGlbPrmVehSpdBilnrSeln  YTbl=HysCmpEffLossY
      settings: AttributesFormatString=Lnr ( u16VariX , u16VariY )
  EffOffsCalc : LnrIntrpn/LnrIntrpn_u16_u16VariXu16VariY  RequirementInfo={'linktype_rmi_doors' '0000a52c (/E-STEER Core/SubSystem Specifications/Application Functions/SF012A Hysteresis Compensation)' '#SF012A_442' 'true' 'REQ:SF012A_442' '' } %GIDa_6c555492_bad9_4001_afb1_b2ea25536550  XTbl=SysGlbPrmVehSpdBilnrSeln  YTbl=HysCmpEffOffsY
      settings: AttributesFormatString=Lnr ( u16VariX , u16VariY )
  FixdToFloat_f32_u1 : FixdToFloat/FixdToFloat_f32_u16  RequirementInfo={'linktype_rmi_doors' '0000a52c (/E-STEER Core/SubSystem Specifications/Application Functions/SF012A Hysteresis Compensation)' '#SF012A_443' 'true' 'REQ:SF012A_443' '' } %GIDa_5cac5b5e_3958_4531_9c71_2690a5a256ad  Param1=12
  FixdToFloat_f32_u16 : FixdToFloat/FixdToFloat_f32_u16  RequirementInfo={'linktype_rmi_doors' '0000a52c (/E-STEER Core/SubSystem Specifications/Application Functions/SF012A Hysteresis Compensation)' '#SF012A_442' 'true' 'REQ:SF012A_442' '' } %GIDa_cab034ab_d6e1_4bfc_88a5_c049e904b751  Param1=7
  FixdToFloat_f32_u2 : FixdToFloat/FixdToFloat_f32_u16  RequirementInfo={'linktype_rmi_doors' '0000a52c (/E-STEER Core/SubSystem Specifications/Application Functions/SF012A Hysteresis Compensation)' '#SF012A_440' 'true' 'REQ:SF012A_440' '' } %GIDa_d7dc8b20_68c8_4a45_adf0_0046cda5bd0c  Param1=7
  FixdToFloat_f32_u3 : FixdToFloat/FixdToFloat_f32_u16  RequirementInfo={'linktype_rmi_doors' '0000a52c (/E-STEER Core/SubSystem Specifications/Application Functions/SF012A Hysteresis Compensation)' '#SF012A_452' 'true' 'REQ:SF012A_452' '' } %GIDa_80ba7869_7fcd_4268_a712_4344b9bc7490  Param1=12
  FixdToFloat_f32_u4 : FixdToFloat/FixdToFloat_f32_u16  RequirementInfo={'linktype_rmi_doors' '0000a52c (/E-STEER Core/SubSystem Specifications/Application Functions/SF012A Hysteresis Compensation)' '#SF012A_453' 'true' 'REQ:SF012A_453' '' } %GIDa_b6b976ce_f5e0_4fc1_bd4c_893be9f8b320  Param1=14
  FixdToFloat_f32_u5 : FixdToFloat/FixdToFloat_f32_u16  RequirementInfo={'linktype_rmi_doors' '0000a52c (/E-STEER Core/SubSystem Specifications/Application Functions/SF012A Hysteresis Compensation)' '#SF012A_453' 'true' 'REQ:SF012A_453' '' } %GIDa_a40e42e5_cc05_4075_99a0_c591098e69ce  Param1=7
  FloatToFixd_u16_f1 : FloatToFixd/FloatToFixd_u16_f32  RequirementInfo={'linktype_rmi_doors' '0000a52c (/E-STEER Core/SubSystem Specifications/Application Functions/SF012A Hysteresis Compensation)' '#SF012A_442' 'true' 'REQ:SF012A_442' '' } %GIDa_c03cc950_f9b0_41c2_9ede_be7e53131c97  Param1=7
  FloatToFixd_u16_f2 : FloatToFixd/FloatToFixd_u16_f32  RequirementInfo={'linktype_rmi_doors' '0000a52c (/E-STEER Core/SubSystem Specifications/Application Functions/SF012A Hysteresis Compensation)' '#SF012A_443' 'true' 'REQ:SF012A_443' '' } %GIDa_4a6315bf_1518_4376_8242_4486d91cbaea  Param1=7
  FloatToFixd_u16_f3 : FloatToFixd/FloatToFixd_u16_f32  RequirementInfo={'linktype_rmi_doors' '0000a52c (/E-STEER Core/SubSystem Specifications/Application Functions/SF012A Hysteresis Compensation)' '#SF012A_440' 'true' 'REQ:SF012A_440' '' } %GIDa_1c2e8502_e46a_4f7a_906a_0a508f33a3f7  Param1=7
  FloatToFixd_u16_f4 : FloatToFixd/FloatToFixd_u16_f32  RequirementInfo={'linktype_rmi_doors' '0000a52c (/E-STEER Core/SubSystem Specifications/Application Functions/SF012A Hysteresis Compensation)' '#SF012A_452' 'true' 'REQ:SF012A_452' '' } %GIDa_820bd048_1267_47ce_bfb2_d50c4f90d68e  Param1=7
  FloatToFixd_u16_f5 : FloatToFixd/FloatToFixd_u16_f32  RequirementInfo={'linktype_rmi_doors' '0000a52c (/E-STEER Core/SubSystem Specifications/Application Functions/SF012A Hysteresis Compensation)' '#SF012A_453' 'true' 'REQ:SF012A_453' '' } %GIDa_47625abf_ede4_4e73_8dde_6e1a215f09a6  Param1=7
  FloatToFixd_u16_f6 : FloatToFixd/FloatToFixd_u16_f32  RequirementInfo={'linktype_rmi_doors' '0000a52c (/E-STEER Core/SubSystem Specifications/Application Functions/SF012A Hysteresis Compensation)' '#SF012A_453' 'true' 'REQ:SF012A_453' '' } %GIDa_00183330_13cf_4979_a8ec_1d09ccb82baa  Param1=8
  FloatToFixd_u16_f7 : FloatToFixd/FloatToFixd_u16_f32  RequirementInfo={'linktype_rmi_doors' '0000a52c (/E-STEER Core/SubSystem Specifications/Application Functions/SF012A Hysteresis Compensation)' '#SF012A_452' 'true' 'REQ:SF012A_452' '' } %GIDa_ac79c81c_7290_47b0_a52f_10b56ac536f1  Param1=12
  HwTqSca : BilnrIntrpnMplX/BilnrIntrpnWithRound_u16_u16MplXu16MplY  RequirementInfo={'linktype_rmi_doors' '0000a52c (/E-STEER Core/SubSystem Specifications/Application Functions/SF012A Hysteresis Compensation)' '#SF012A_452' 'true' 'REQ:SF012A_452' '' } %GIDa_94008122_b415_4e33_afaa_9cd5d0edffee  MplXTbl=HysCmpHwTqScaX  MplYTbl=HysCmpHwTqScaY  BilnrSelnTbl=SysGlbPrmVehSpdBilnrSeln
      settings: AttributesFormatString=Bilnr ( u16MplX , u16MplY )
  HysSatn : LnrIntrpn/LnrIntrpn_u16_u16VariXu16VariY  RequirementInfo={'linktype_rmi_doors' '0000a52c (/E-STEER Core/SubSystem Specifications/Application Functions/SF012A Hysteresis Compensation)' '#SF012A_440' 'true' 'REQ:SF012A_440' '' } %GIDa_28146c01_6696_4f34_be63_bf58a35c604b  XTbl=SysGlbPrmVehSpdBilnrSeln  YTbl=HysCmpHysSatnY
      settings: AttributesFormatString=Lnr ( u16VariX , u16VariY )
  Max_f32 : NxtrMax/Max_f32  RequirementInfo={'linktype_rmi_doors' '0000a52c (/E-STEER Core/SubSystem Specifications/Application Functions/SF012A Hysteresis Compensation)' '#SF012A_442' 'true' 'REQ:SF012A_442' '' } %GIDa_ae37927a_b75d_4e0b_8fda_ff88938a69ba  SFunctionSpec=single y1 = Max_f32(single u1, single u2)
      settings: AttributesFormatString=%<Name>
  NegHysCmp : LnrIntrpn/LnrIntrpn_u16_u16VariXu16VariY  RequirementInfo={'linktype_rmi_doors' '0000a52c (/E-STEER Core/SubSystem Specifications/Application Functions/SF012A Hysteresis Compensation)' '#SF012A_453' 'true' 'REQ:SF012A_453' '' } %GIDa_8f2684a9_9f6c_419a_9d72_6a02b2a00374  XTbl=HysCmpNegHysCmpX  YTbl=HysCmpNegHysCmpY
      settings: AttributesFormatString=Lnr ( u16VariX , u16VariY )
  NegHysCmpSca : LnrIntrpn/LnrIntrpn_u16_u16VariXu16VariY  RequirementInfo={'linktype_rmi_doors' '0000a52c (/E-STEER Core/SubSystem Specifications/Application Functions/SF012A Hysteresis Compensation)' '#SF012A_453' 'true' 'REQ:SF012A_453' '' } %GIDa_d3aee8be_a43c_401f_be49_356fe935243d  XTbl=HysCmpNegHysCmpScaX  YTbl=HysCmpNegHysCmpScaY
      settings: AttributesFormatString=Lnr ( u16VariX , u16VariY )
  Product : Product  RequirementInfo={'linktype_rmi_doors' '0000a52c (/E-STEER Core/SubSystem Specifications/Application Functions/SF012A Hysteresis Compensation)' '#SF012A_452' 'true' 'REQ:SF012A_452' '' } %GIDa_849eebbf_f800_40fc_aeba_72544c049dcc  RndMeth=Zero
  Product1 : Product  RequirementInfo={'linktype_rmi_doors' '0000a52c (/E-STEER Core/SubSystem Specifications/Application Functions/SF012A Hysteresis Compensation)' '#SF012A_443' 'true' 'REQ:SF012A_443' '' } %GIDa_0fa58c1b_05e1_4572_8dfb_8ac09a260d67  RndMeth=Zero
  Product2 : Product  RequirementInfo={'linktype_rmi_doors' '0000a52c (/E-STEER Core/SubSystem Specifications/Application Functions/SF012A Hysteresis Compensation)' '#SF012A_453' 'true' 'REQ:SF012A_453' '' } %GIDa_4a13052a_ae74_4fe4_935a_4d1ecab5c2e7  RndMeth=Zero
  Satn : NxtrLim/LimDyn_f32  RequirementInfo={'linktype_rmi_doors' '0000a52c (/E-STEER Core/SubSystem Specifications/Application Functions/SF012A Hysteresis Compensation)' '#SF012A_440' 'true' 'REQ:SF012A_440' '' } %GIDa_f42743cd_68e7_45cd_9233_f0f945e15772
  CmpAvl : Outport  RequirementInfo={'linktype_rmi_doors' '0000a52c (/E-STEER Core/SubSystem Specifications/Application Functions/SF012A Hysteresis Compensation)' '#SF012A_438' 'true' 'REQ:SF012A_438' '' ; 'linktype_rmi_doors' '0000a52c (/E-STEER Core/SubSystem Specifications/Application Functions/SF012A Hysteresis Compensation)' '#SF012A_454' 'true' 'REQ:SF012A_454' '' } %GIDa_72df7f48_3f77_4521_8683_9aa1cb528292
  wires:
  AssiCmdFild/1 -> [AssiCmdFild]
  VehSpd/1 -> [VehSpd]
  HwTqFild/1 -> [HwTqFild]
  WhlImbRejctnAmp/1 -> [WhlImbRejctnAmp]
  [HwTqFild] -> Add1/1
  [AssiCmdFild] -> Add1/2
  Add1/1 -> Abslt_f32_f32/1
  [VehSpd] -> FloatToFixd_u16_f1/1
  Abslt_f32_f32/1 -> Add2/1
  EffOffsCalc/1 -> FixdToFloat_f32_u16/1
  Add2/1 -> Max_f32/1
  Constant2/1 -> Max_f32/2
  [VehSpd] -> FloatToFixd_u16_f2/1
  EffLossCalc/1 -> FixdToFloat_f32_u1/1
  FloatToFixd_u16_f1/1 -> EffOffsCalc/1
  FixdToFloat_f32_u16/1 -> Add2/2
  FloatToFixd_u16_f2/1 -> EffLossCalc/1
  FixdToFloat_f32_u1/1 -> Product1/2
  AssiMechT/1 -> CoulombFric/1(AssiMechT)
  [VehSpd] -> CoulombFric/3(VehSpd)
  SysFricOffs/1 -> CoulombFric/2(SysFricOffs)
  [WhlImbRejctnAmp] -> CoulombFric/4(WhlImbRejctnAmp)
  Product1/1 -> Add3/1, Data Store Write1/1  "HysCmpEffCmpTq"
  CoulombFric/1(CoulombFric) -> Add3/2  "CoulombFric"
  Add3/1 -> Satn/1  "HysTqNotLimd"
  Constant1/1 -> Satn/2
  HysSatn/1 -> FixdToFloat_f32_u2/1
  [VehSpd] -> FloatToFixd_u16_f3/1
  FloatToFixd_u16_f3/1 -> HysSatn/1
  FixdToFloat_f32_u2/1 -> Satn/3
  Satn/1 -> [HysTq]
  [HysTq] -> Product/1
  [HwTqFild] -> Abslt_f32_f1/1
  Abslt_f32_f1/1 -> FloatToFixd_u16_f7/1
  [VehSpd] -> FloatToFixd_u16_f4/1
  HwTqSca/1 -> FixdToFloat_f32_u3/1
  FloatToFixd_u16_f4/1 -> HwTqSca/2
  Product/1 -> Data Store Write4/1, Add4/1
  [AssiCmdFild] -> Abslt_f32_f2/1
  Abslt_f32_f2/1 -> FloatToFixd_u16_f5/1
  FloatToFixd_u16_f5/1 -> NegHysCmpSca/1
  FixdToFloat_f32_u3/1 -> Product/2
  NegHysCmpSca/1 -> FixdToFloat_f32_u4/1
  FixdToFloat_f32_u4/1 -> Product2/1
  [WhlImbRejctnAmp] -> FloatToFixd_u16_f6/1
  FloatToFixd_u16_f6/1 -> NegHysCmp/1
  NegHysCmp/1 -> FixdToFloat_f32_u5/1
  FixdToFloat_f32_u5/1 -> Product2/2
  Product2/1 -> Data Store Write2/1, Add4/2
  Add4/1 -> Data Store Write3/1, CmpAvl/1
  Max_f32/1 -> Product1/1
  FloatToFixd_u16_f7/1 -> HwTqSca/1

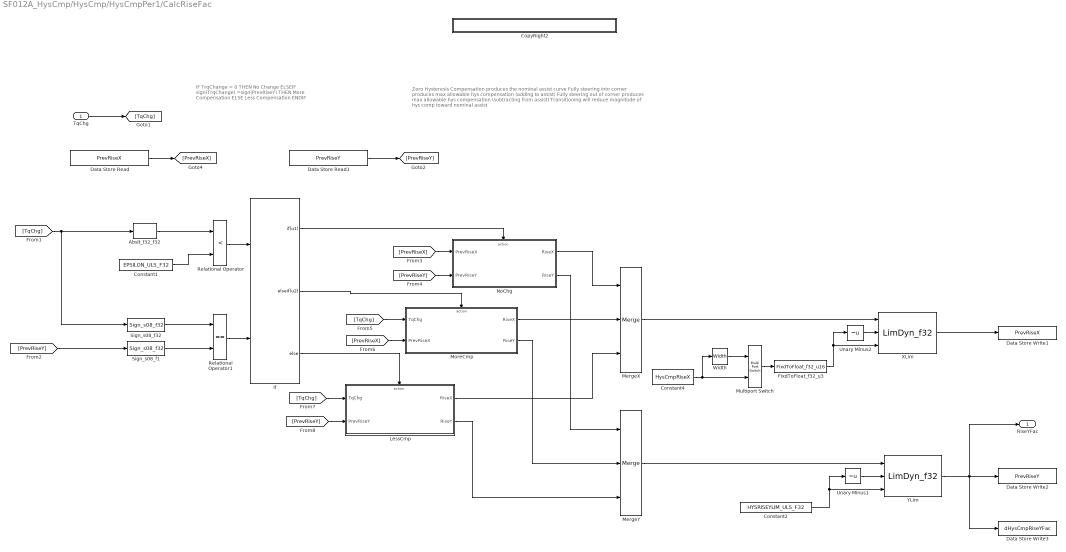
== system SF012A_HysCmp/HysCmp/HysCmpPer1/CalcRiseFac ==
  note: IF TrqChange = 0  THEN
      |      No Change
      | ELSEIF sign(TrqChange) =sign(PrevRiseY)  THEN
      |      More Compensation
      | ELSE
      |      Less Compensation
      | ENDIF
  note: Zero Hysteresis Compensation produces the nominal assist curve
      | Fully steering into corner produces max allowable hys compensation (adding to assist)
      | Fully steering out of corner produces max allowable hys compensation (subtracting from assist)
      | Transitioning will reduce magnitude of hys comp toward nominal assist
  TqChg : Inport
  Abslt_f32_f32 : NxtrAbslt/Abslt_f32_f32  RequirementInfo={'linktype_rmi_doors' '0000a52c (/E-STEER Core/SubSystem Specifications/Application Functions/SF012A Hysteresis Compensation)' '#SF012A_420' 'true' 'REQ:SF012A_420' '' ; 'linktype_rmi_doors' '0000a52c (/E-STEER Core/SubSystem Specifications/Application Functions/SF012A Hysteresis Compensation)' '#SF012A_421' 'true' 'REQ:SF012A_421' '' ; 'linktype_rmi_doors' '0000a52c (/E-STEER Core/SubSystem Specifications/Application Functions/SF012A Hysteresis Compensation)' '#SF012A_428' 'true' 'REQ:SF012A_428' '' } %GIDa_00ebcca8_adc1_46d3_9272_20e617ef8354  SFunctionSpec=single y1 = Abslt_f32_f32(single u1)
      settings: AttributesFormatString=%<Name>
  Constant1 : Constant  RequirementInfo={'linktype_rmi_doors' '0000a52c (/E-STEER Core/SubSystem Specifications/Application Functions/SF012A Hysteresis Compensation)' '#SF012A_420' 'true' 'REQ:SF012A_420' '' ; 'linktype_rmi_doors' '0000a52c (/E-STEER Core/SubSystem Specifications/Application Functions/SF012A Hysteresis Compensation)' '#SF012A_421' 'true' 'REQ:SF012A_421' '' ; 'linktype_rmi_doors' '0000a52c (/E-STEER Core/SubSystem Specifications/Application Functions/SF012A Hysteresis Compensation)' '#SF012A_428' 'true' 'REQ:SF012A_428' '' } %GIDa_281f4ec9_cf01_48c4_8e2d_5232a3f65859  Value=EPSILON_ULS_F32
  Constant2 : Constant  RequirementInfo={'linktype_rmi_doors' '0000a52c (/E-STEER Core/SubSystem Specifications/Application Functions/SF012A Hysteresis Compensation)' '#SF012A_416' 'true' 'REQ:SF012A_416' '' } %GIDa_dccac7b9_47c9_4dc3_8bf2_c5841d6162d3  Value=HYSRISEYLIM_ULS_F32
  Constant4 : Constant  RequirementInfo={'linktype_rmi_doors' '0000a52c (/E-STEER Core/SubSystem Specifications/Application Functions/SF012A Hysteresis Compensation)' '#SF012A_418' 'true' 'REQ:SF012A_418' '' } %GIDa_67a40d73_9937_4a74_9c18_2a5c9262c575  Value=HysCmpRiseX
  CopyRight2 : Subsystem  Description=|  mask(Copyright Information){none=on}
      | Copyright info block.                                               
      |                                                                     
      | Place copyright information at the top of every subsystem in design.
      mask prompts: none "No parameters"
      mask help: Place copyright information at the top of every subsystem in design.
      mask Display:
      | NxtrConf = 'Nexteer Confidential';
      | 
      | sys = bdroot; %handle for the current model ("system")
      | first = get_param(sys,'Created');
      | if(isempty(first))
      |     first = datestr(now,'yyyy');
      | else
      |     first = first(end-3:end);  %year is last four digits
      | end
      | 
      | last = get_param(sys,'LastModifiedDate');
      | if isempty(last)
      |     last = datestr(now,'yyyy');
      | else
      |     last = last(end-3:end);
      | end
      | 
      | if strcmp(first,last)
      |     fprintf('%s -- Copyright %s Nexteer',NxtrConf,first)
      | else
      |     fprintf('%s -- %s%s- %s Nexteer',NxtrConf,char(169),first,last)
      | end
  Data Store Read : DataStoreRead  DataStoreName=PrevRiseX
  Data Store Read1 : DataStoreRead  DataStoreName=PrevRiseY
  Data Store Write1 : DataStoreWrite  RequirementInfo={'linktype_rmi_doors' '0000a52c (/E-STEER Core/SubSystem Specifications/Application Functions/SF012A Hysteresis Compensation)' '#SF012A_417' 'true' 'REQ:SF012A_417' '' } %GIDa_79abe55e_0d9f_4f5a_affd_f80280fe4806  DataStoreName=PrevRiseX
  Data Store Write2 : DataStoreWrite  DataStoreName=PrevRiseY
  Data Store Write3 : DataStoreWrite  DataStoreName=dHysCmpRiseYFac
  FixdToFloat_f32_u3 : FixdToFloat/FixdToFloat_f32_u16  RequirementInfo={'linktype_rmi_doors' '0000a52c (/E-STEER Core/SubSystem Specifications/Application Functions/SF012A Hysteresis Compensation)' '#SF012A_418' 'true' 'REQ:SF012A_418' '' } %GIDa_eb58a2f0_0921_4335_8581_1b09fc1b9188  Param1=14
  If : If  RequirementInfo={'linktype_rmi_doors' '0000a52c (/E-STEER Core/SubSystem Specifications/Application Functions/SF012A Hysteresis Compensation)' '#SF012A_421' 'true' 'REQ:SF012A_421' '' ; 'linktype_rmi_doors' '0000a52c (/E-STEER Core/SubSystem Specifications/Application Functions/SF012A Hysteresis Compensation)' '#SF012A_423' 'true' 'REQ:SF012A_423' '' ; 'linktype_rmi_doors' '0000a52c (/E-STEER Core/SubSystem Specifications/Application Functions/SF012A Hysteresis Compensation)' '#SF012A_428' 'true' 'REQ:SF012A_428' '' } %GIDa_58cce5e2_fc42_4d32_9d8c_52d5a58d4b35  NumInputs=2  IfExpression=u1  ElseIfExpressions=u2
  LessCmp : Subsystem  RequirementInfo={'linktype_rmi_doors' '0000a52c (/E-STEER Core/SubSystem Specifications/Application Functions/SF012A Hysteresis Compensation)' '#SF012A_426' 'true' 'REQ:SF012A_426' '' } %GIDa_c6d0ce65_cc69_4af1_8323_e14a01f9295b  TreatAsAtomicUnit=on
  MergeX : Merge  Inputs=3
  MergeY : Merge  Inputs=3
  MoreCmp : Subsystem  RequirementInfo={'linktype_rmi_doors' '0000a52c (/E-STEER Core/SubSystem Specifications/Application Functions/SF012A Hysteresis Compensation)' '#SF012A_422' 'true' 'REQ:SF012A_422' '' } %GIDa_4ce48d41_d7e0_4702_8f37_cf1925e87b2c  TreatAsAtomicUnit=on
  Multiport Switch : MultiPortSwitch  RequirementInfo={'linktype_rmi_doors' '0000a52c (/E-STEER Core/SubSystem Specifications/Application Functions/SF012A Hysteresis Compensation)' '#SF012A_418' 'true' 'REQ:SF012A_418' '' } %GIDa_b814a708_c3c4_46cb_aded_5a29f105308e  Inputs=1
  NoChg : Subsystem  RequirementInfo={'linktype_rmi_doors' '0000a52c (/E-STEER Core/SubSystem Specifications/Application Functions/SF012A Hysteresis Compensation)' '#SF012A_420' 'true' 'REQ:SF012A_420' '' ; 'linktype_rmi_doors' '0000a52c (/E-STEER Core/SubSystem Specifications/Application Functions/SF012A Hysteresis Compensation)' '#SF012A_421' 'true' 'REQ:SF012A_421' '' ; 'linktype_rmi_doors' '0000a52c (/E-STEER Core/SubSystem Specifications/Application Functions/SF012A Hysteresis Compensation)' '#SF012A_419' 'true' 'REQ:SF012A_419' '' } %GIDa_415a6946_680d_47a8_bfef_3603d26400f6  TreatAsAtomicUnit=on
  Relational Operator : RelationalOperator  RequirementInfo={'linktype_rmi_doors' '0000a52c (/E-STEER Core/SubSystem Specifications/Application Functions/SF012A Hysteresis Compensation)' '#SF012A_420' 'true' 'REQ:SF012A_420' '' ; 'linktype_rmi_doors' '0000a52c (/E-STEER Core/SubSystem Specifications/Application Functions/SF012A Hysteresis Compensation)' '#SF012A_421' 'true' 'REQ:SF012A_421' '' ; 'linktype_rmi_doors' '0000a52c (/E-STEER Core/SubSystem Specifications/Application Functions/SF012A Hysteresis Compensation)' '#SF012A_428' 'true' 'REQ:SF012A_428' '' } %GIDa_cbebcd3e_31e6_4f12_8917_002a18af1d2e  Operator=<  OutDataTypeStr=boolean
  Relational Operator1 : RelationalOperator  RequirementInfo={'linktype_rmi_doors' '0000a52c (/E-STEER Core/SubSystem Specifications/Application Functions/SF012A Hysteresis Compensation)' '#SF012A_423' 'true' 'REQ:SF012A_423' '' ; 'linktype_rmi_doors' '0000a52c (/E-STEER Core/SubSystem Specifications/Application Functions/SF012A Hysteresis Compensation)' '#SF012A_428' 'true' 'REQ:SF012A_428' '' } %GIDa_c021790f_f358_4ec0_9a4c_252a83e43cf0  Operator===  OutDataTypeStr=boolean
  Sign_s08_f1 : NxtrSign/Sign_s08_f32  RequirementInfo={'linktype_rmi_doors' '0000a52c (/E-STEER Core/SubSystem Specifications/Application Functions/SF012A Hysteresis Compensation)' '#SF012A_423' 'true' 'REQ:SF012A_423' '' ; 'linktype_rmi_doors' '0000a52c (/E-STEER Core/SubSystem Specifications/Application Functions/SF012A Hysteresis Compensation)' '#SF012A_428' 'true' 'REQ:SF012A_428' '' } %GIDa_f253b20a_f1ca_4c8b_a0d6_2544ed91ce70  SFunctionSpec=int8 y1 = Sign_s08_f32(single u1)
  Sign_s08_f32 : NxtrSign/Sign_s08_f32  RequirementInfo={'linktype_rmi_doors' '0000a52c (/E-STEER Core/SubSystem Specifications/Application Functions/SF012A Hysteresis Compensation)' '#SF012A_423' 'true' 'REQ:SF012A_423' '' ; 'linktype_rmi_doors' '0000a52c (/E-STEER Core/SubSystem Specifications/Application Functions/SF012A Hysteresis Compensation)' '#SF012A_428' 'true' 'REQ:SF012A_428' '' } %GIDa_b723e255_145a_469d_8eed_bc23d4eb85d7  SFunctionSpec=int8 y1 = Sign_s08_f32(single u1)
  Unary Minus1 : UnaryMinus  RequirementInfo={'linktype_rmi_doors' '0000a52c (/E-STEER Core/SubSystem Specifications/Application Functions/SF012A Hysteresis Compensation)' '#SF012A_416' 'true' 'REQ:SF012A_416' '' } %GIDa_9a52ea14_be8b_4ff6_9bcc_24e4239b4911
  Unary Minus2 : UnaryMinus  RequirementInfo={'linktype_rmi_doors' '0000a52c (/E-STEER Core/SubSystem Specifications/Application Functions/SF012A Hysteresis Compensation)' '#SF012A_418' 'true' 'REQ:SF012A_418' '' } %GIDa_61f988a7_3450_4f52_9543_7649dcf33eba
  Width : Width  RequirementInfo={'linktype_rmi_doors' '0000a52c (/E-STEER Core/SubSystem Specifications/Application Functions/SF012A Hysteresis Compensation)' '#SF012A_418' 'true' 'REQ:SF012A_418' '' } %GIDa_26449ae7_c65d_4b33_93d2_dbb66589b586  DataType=uint16
  XLim : NxtrLim/LimDyn_f32  RequirementInfo={'linktype_rmi_doors' '0000a52c (/E-STEER Core/SubSystem Specifications/Application Functions/SF012A Hysteresis Compensation)' '#SF012A_418' 'true' 'REQ:SF012A_418' '' } %GIDa_74a422c5_7f6d_47c8_89e4_98d9e21c5f4e
  YLim : NxtrLim/LimDyn_f32  RequirementInfo={'linktype_rmi_doors' '0000a52c (/E-STEER Core/SubSystem Specifications/Application Functions/SF012A Hysteresis Compensation)' '#SF012A_416' 'true' 'REQ:SF012A_416' '' } %GIDa_192879d9_a019_4c77_aaad_dc1543fb4578
  RiseYFac : Outport  RequirementInfo={'linktype_rmi_doors' '0000a52c (/E-STEER Core/SubSystem Specifications/Application Functions/SF012A Hysteresis Compensation)' '#SF012A_415' 'true' 'REQ:SF012A_415' '' } %GIDa_a7f07ddd_5ea4_4fe1_9b53_1d462caa880e
  wires:
  Sign_s08_f1/1 -> Relational Operator1/2
  If/2 -> MoreCmp/Action
  If/3 -> LessCmp/Action
  [TqChg] -> Sign_s08_f32/1, Abslt_f32_f32/1
  Sign_s08_f32/1 -> Relational Operator1/1
  If/1 -> NoChg/Action
  TqChg/1 -> [TqChg]
  NoChg/1(RiseX) -> MergeX/1
  MoreCmp/1(RiseX) -> MergeX/2
  LessCmp/1(RiseX) -> MergeX/3
  NoChg/2(RiseY) -> MergeY/1
  MoreCmp/2(RiseY) -> MergeY/2
  LessCmp/2(RiseY) -> MergeY/3
  MergeX/1 -> XLim/1
  MergeY/1 -> YLim/1
  FixdToFloat_f32_u3/1 -> XLim/3, Unary Minus2/1
  Unary Minus2/1 -> XLim/2
  Unary Minus1/1 -> YLim/2
  Data Store Read/1 -> [PrevRiseX]
  Data Store Read1/1 -> [PrevRiseY]
  [PrevRiseY] -> Sign_s08_f1/1
  [PrevRiseX] -> NoChg/1(PrevRiseX)
  [PrevRiseY] -> NoChg/2(PrevRiseY)
  [TqChg] -> MoreCmp/1(TqChg)
  [PrevRiseX] -> MoreCmp/2(PrevRiseX)
  [TqChg] -> LessCmp/1(TqChg)
  [PrevRiseY] -> LessCmp/2(PrevRiseY)
  Constant4/1 -> Multiport Switch/2, Width/1
  Width/1 -> Multiport Switch/1
  Multiport Switch/1 -> FixdToFloat_f32_u3/1
  YLim/1 -> Data Store Write3/1, Data Store Write2/1, RiseYFac/1
  XLim/1 -> Data Store Write1/1
  Constant2/1 -> YLim/3, Unary Minus1/1
  Relational Operator/1 -> If/1
  Abslt_f32_f32/1 -> Relational Operator/1
  Constant1/1 -> Relational Operator/2
  Relational Operator1/1 -> If/2

== system SF012A_HysCmp/HysCmp/HysCmpPer1/CopyRight2 ==
